simulink model "lpa1_SIL_harness"  (R2024a)
settings: Solver=FixedStepDiscrete  StartTime=0.0  StopTime=6  FixedStep=0.01  RelTol=1e-3
undefined symbols (not defined in the file): DiscIntNeverNeededParam
settings Model: SILPILSystemUnderTest=refmodels  SILPILSimulationModeModelRef=accelerator  Creator=Anas  LastModifiedBy=Anas
settings OptimizationCC: DefaultParameterBehavior=Inlined  EnhancedBackFolding=on  PassReuseOutputArgsAs=Individual arguments  ZeroExternalMemoryAtStartup=off  ZeroInternalMemoryAtStartup=off  OptimizeBlockOrder=speed  DifferentSizesBufferReuse=on  OptimizationCustomize=off  EfficientTunableParamExpr=on
settings DebuggingCC: ParameterTunabilityLossMsg=error
settings SFSimCC: MATLABDynamicMemAlloc=off
settings RTWCC: Description=Embedded Coder  SystemTargetFile=ert.tlc  TemplateMakefile=ert_default_tmf  Toolchain=MinGW64 | gmake (64-bit Windows)
settings CodeAppCC: ForceParamTrailComments=on  IgnoreCustomStorageClasses=off  OperatorAnnotations=on  SimulinkDataObjDesc=on  SFDataObjDesc=on  InsertBlockDesc=on
settings ERTTargetCC: TargetLangStandard=C99 (ISO)  GenerateSampleERTMain=on  InlinedParameterPlacement=NonHierarchical  ERTCustomFileTemplate=example_file_process.tlc
settings ConfigComp: CovEnable=on  RecordCoverage=on  CovMetricSettings=dcmwe  CovModelRefEnable=on  DVTestSuiteOptimization=Auto  DVDetectOutOfBounds=on  DVModelReferenceHarness=on  DVHarnessSource=Signal Editor

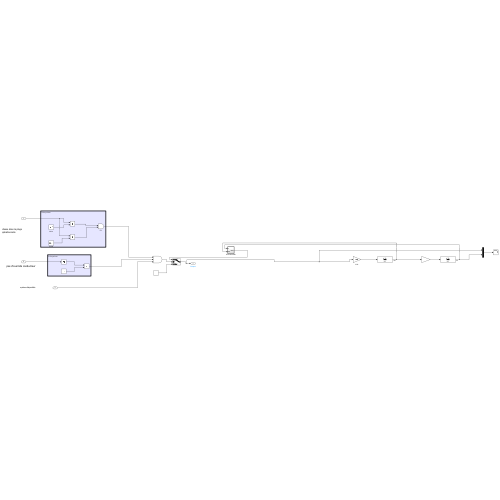
[thumbnail: Simulink's stored preview of the top-level diagram]
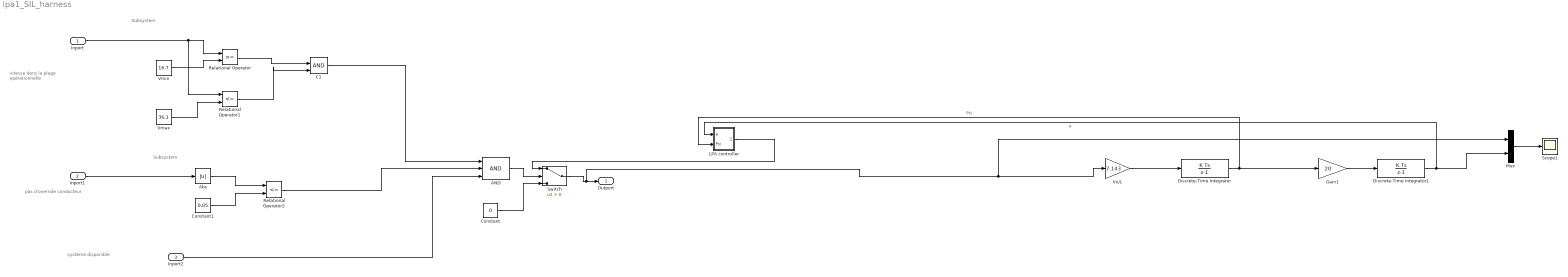
== system lpa1_SIL_harness ==
  note: système disponible
  note: pas d'override conducteur
  note: vitesse dans la plage opérationnelle
  note: Subsystem
  note: Subsystem
  Inport : Inport
  Inport1 : Inport  Port=2
  Inport2 : Inport  Port=3
  AND : Logic  Inputs=3  IconShape=distinctive  AllPortsSameDT=off  OutDataTypeStr=boolean
  Abs : Abs  SaturateOnIntegerOverflow=off
  C1 : Logic  IconShape=distinctive  AllPortsSameDT=off  OutDataTypeStr=boolean
  Constant : Constant  Value=0
  Constant1 : Constant  Value=0.05
  Discrete-Time Integrator : DiscreteIntegrator  SampleTime=0.01  ICPrevOutput=DiscIntNeverNeededParam  ICPrevScaledInput=DiscIntNeverNeededParam
  Discrete-Time Integrator1 : DiscreteIntegrator  InitialCondition=0.5  SampleTime=0.01  ICPrevOutput=DiscIntNeverNeededParam  ICPrevScaledInput=DiscIntNeverNeededParam
  Gain1 : Gain  Gain=20
  LPA controller : Subsystem  TreatAsAtomicUnit=on  SystemSampleTime=0.01
  Mux : Mux  Inputs=2
  Relational Operator : RelationalOperator  OutDataTypeStr=boolean  RndMeth=Simplest  InputSameDT=off
  Relational Operator1 : RelationalOperator  Operator=<=  OutDataTypeStr=boolean  RndMeth=Simplest  InputSameDT=off
  Relational Operator2 : RelationalOperator  Operator=<=  OutDataTypeStr=boolean  RndMeth=Simplest  InputSameDT=off
  Scope1 : Scope
  Switch : Switch  Criteria=u2 > Threshold  SaturateOnIntegerOverflow=off  InputSameDT=off
  Vmax : Constant  Value=36.1
  Vmin : Constant  Value=16.7
  Vx/L : Gain  Gain=7.143
  Outport : Outport
  wires:
  Vx/L/1 -> Discrete-Time Integrator/1
  Discrete-Time Integrator/1 -> LPA controller/2(Psi), Gain1/1  "Psi"
  Gain1/1 -> Discrete-Time Integrator1/1
  Discrete-Time Integrator1/1 -> LPA controller/1(e), Mux/2  "e"
  Mux/1 -> Scope1/1
  LPA controller/1(delta) -> Switch/1
  AND/1 -> Switch/2
  Constant/1 -> Switch/3
  C1/1 -> AND/1
  Vmin/1 -> Relational Operator/2
  Relational Operator/1 -> C1/1
  Vmax/1 -> Relational Operator1/2
  Relational Operator1/1 -> C1/2
  Inport/1 -> Relational Operator1/1, Relational Operator/1
  Relational Operator2/1 -> AND/2
  Inport1/1 -> Abs/1
  Constant1/1 -> Relational Operator2/2
  Abs/1 -> Relational Operator2/1
  Inport2/1 -> AND/3
  Switch/1 -> Mux/1, Vx/L/1, Outport/1

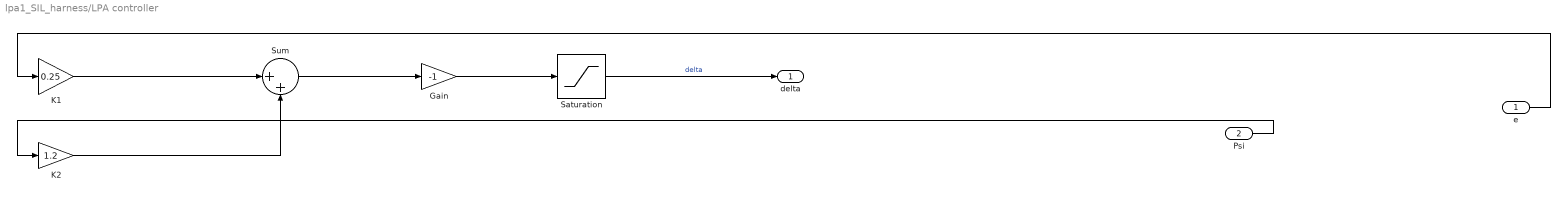
== system lpa1_SIL_harness/LPA controller ==
  e : Inport
  Psi : Inport  Port=2
  Gain : Gain  Gain=-1
  K1 : Gain  Gain=0.25
  K2 : Gain  Gain=1.2
  Saturation : Saturate
  Sum : Sum  Inputs=|++
  delta : Outport
  wires:
  Sum/1 -> Gain/1
  K1/1 -> Sum/1
  Gain/1 -> Saturation/1
  e/1 -> K1/1
  K2/1 -> Sum/2
  Saturation/1 -> delta/1  "delta"
  Psi/1 -> K2/1
